simulink model "Linea2DF"  (R2022b)
settings: Solver=VariableStepAuto  StartTime=0.0  StopTime=50  RelTol=1e-3
settings Model: Creator=ASOAT  LastModifiedBy=ASOAT

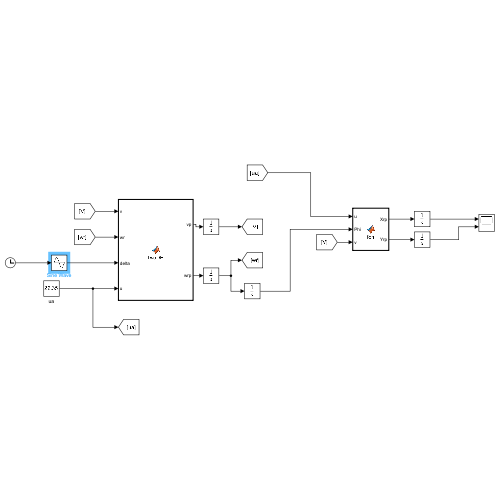
[thumbnail: Simulink's stored preview of the top-level diagram]
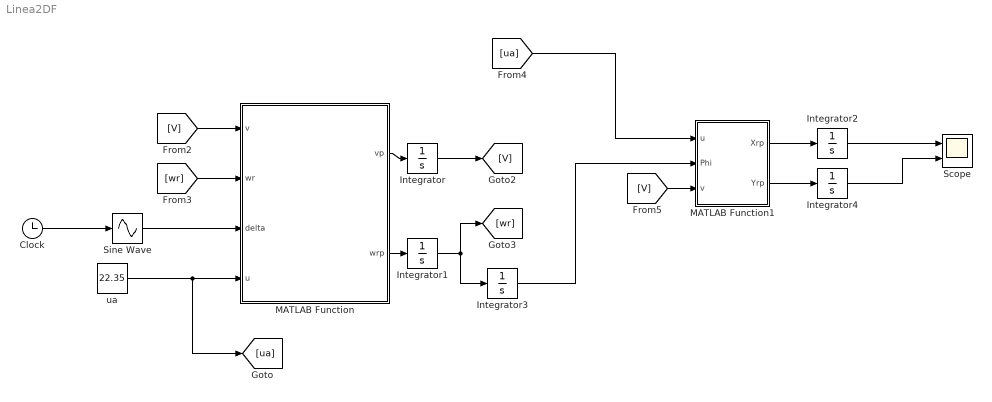
== system Linea2DF ==
  Clock : Clock
  Integrator{,1..4} (5 alike) : Integrator
  MATLAB Function : MATLAB Function  TreatAsAtomicUnit=on
  MATLAB Function1 : MATLAB Function  TreatAsAtomicUnit=on
  Scope : Scope  NumInputPorts=2
  Sine Wave : Sin  TimeSource=Use external signal  Amplitude=pi/6  SampleTime=0
  ua : Constant  Value=22.35
  wires:
  MATLAB Function/1(vp) -> Integrator/1
  MATLAB Function/2(wrp) -> Integrator1/1
  [V] -> MATLAB Function/1(v)
  [wr] -> MATLAB Function/2(wr)
  [ua] -> MATLAB Function1/1(u)
  Integrator/1 -> [V]
  Integrator1/1 -> Integrator3/1, [wr]
  MATLAB Function1/1(Xrp) -> Integrator2/1
  MATLAB Function1/2(Yrp) -> Integrator4/1
  Integrator2/1 -> Scope/1
  Integrator4/1 -> Scope/2
  Integrator3/1 -> MATLAB Function1/2(Phi)
  [V] -> MATLAB Function1/3(v)
  ua/1 -> [ua], MATLAB Function/4(u)
  Sine Wave/1 -> MATLAB Function/3(delta)
  Clock/1 -> Sine Wave/1

== matlab function Linea2DF/MATLAB Function1 ==
  data: u input; Xrp output; Phi input; Yrp output; v input
function [Xrp, Yrp] = fcn(u,Phi,v)

beta = atan(v/u);

gamma = beta + Phi;


Xrp = cos(gamma)*u;
Yrp = sin(gamma)*u;

== matlab function Linea2DF/MATLAB Function ==
  data: v input; wr input; delta input; vp output; wrp output; u input
function [vp,wrp] =  twoDF(v, wr,delta,u)
m = 1818.2;
Iz = 3885;
a = 1.463;
b = 1.585;
k1 = -62618;
k2 = -110185;

vp = ((k1+k2)*v/u+(1/u)*(a*k1-b*k2)*wr-k1*delta)/m - u*wr;
wrp = ((a*k1-b*k2)*v/u+(1/u)*(a^2*k1+b^2*k2)*wr-a*k1*delta)/Iz;
